simulink model "sar_adc_3"  (R2018a)
settings: Solver=ode23tb  StartTime=0.0  StopTime=1e-3  MaxStep=.5/ADC_clock  RelTol=1e-3  EnableMultiTasking=on
InitFcn:
  | % General Parameters
  | Nbits=12;
  | Fs=5e7;      % ADC conversion rate
  | ADC_clock = Fs*(Nbits+2); % required clock rate
  | 
  | 
  | % DAC parameters
  | Vref=2*sqrt(2);   % DAC voltage reference
  | Ron=100;             % switch on resistance
  | C=0.3e-12;           % unit capacitor
  | 
  | % Test Source Parameters
  | A1=Vref/4; A2=A1;   % amplitudes
  | F1=16*Fs/128;           % frequency
  | F2=18*Fs/128;
libraries: powerlib x64, simulink x26
settings Model: SimulationMode=accelerator  Creator=Dick  LastModifiedBy=lenovo
settings SolverCC: ZeroCrossControl=EnableAll  AlgebraicLoopSolver=LineSearch
settings DataIOCC: LimitDataPoints=on  SaveFormat=Array  SignalLoggingSaveFormat=ModelDataLogs
settings OptimizationCC: ExpressionDepthLimit=2147483647  LifeSpan=inf
settings DebuggingCC: UnderspecifiedInitializationDetection=Classic  MergeDetectMultiDrivingBlocksExec=none  SolverPrmCheckMsg=warning  ParameterPrecisionLossMsg=none  FcnCallInpInsideContextMsg=warning  StateNameClashWarn=warning  SFUnexpectedBacktrackingDiag=warning  SFNoUnconditionalDefaultTransitionDiag=warning  SFExecutionAtInitializationDiag=none
settings HardwareCC: ProdBitPerPointer=32  ProdBitPerSizeT=32  ProdBitPerPtrDiffT=32  ProdLargestAtomicFloat=None  ProdIntDivRoundTo=Undefined  ProdEndianess=Unspecified  ProdWordSize=32  ProdHWDeviceType=32-bit Generic
settings ModelReferenceCC: PropagateSignalLabelsOutOfModel=off
settings SFSimCC: SimParseCustomCode=off
settings CodeAppCC: StateflowObjectComments=on
settings GRTTargetCC: TargetLangStandard=C89/C90 (ANSI)  GeneratePreprocessorConditionals=Disable all  CombineOutputUpdateFcns=off  GRTInterface=on
settings ConfigComp: CovMetricSettings=dw  CovHtmlReporting=on  CovSaveCumulativeToWorkspaceVar=on  CovSaveSingleToWorkspaceVar=on  CovExternalEMLEnable=off  CovSFcnEnable=off
settings SimscapeCC: EditingMode=Restricted  SimscapeNormalizeSystem=off

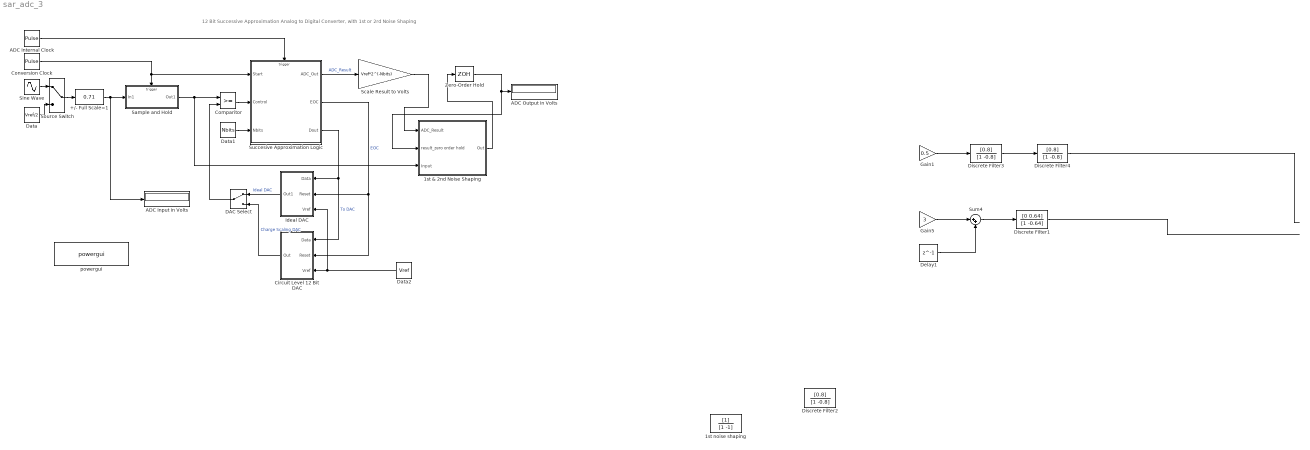
== system sar_adc_3 ==
  note: 12 Bit Successive Approximation Analog to Digital Converter, with 1st or 2rd Noise Shaping
  +/- Full Scale=1 : simulink/Math Operations/Slider Gain  gain=0.71  low=-1  high=1
  1st & 2nd Noise Shaping : Subsystem
  1st noise shaping : DiscreteFilter  Denominator=[1 -1]
  ADC Input in Volts : Display
      settings: Decimation=1000
  ADC Internal Clock : DiscretePulseGenerator  PulseType=Time based  Period=1/ADC_clock  PulseWidth=5
  ADC Output in Volts : Display
      settings: Decimation=1000
  Circuit Level 12 Bit DAC : Subsystem
  Comparitor : RelationalOperator  OutDataTypeStr=boolean  RndMeth=Nearest
  Conversion Clock : DiscretePulseGenerator  PulseType=Time based  Period=1/Fs  PulseWidth=5
  DAC Select : ManualSwitch
  Data : Constant  Value=Vref/2
  Data1 : Constant  Value=Nbits
  Data2 : Constant  Value=Vref
  Delay1 : Delay  DelayLength=1
  Discrete Filter1 : DiscreteFilter  Numerator=[0 0.64]  Denominator=[1 -0.64]
  Discrete Filter2 : DiscreteFilter  Numerator=[0.8]  Denominator=[1 -0.8]
  Discrete Filter3 : DiscreteFilter  Numerator=[0.8]  Denominator=[1 -0.8]
  Discrete Filter4 : DiscreteFilter  Numerator=[0.8]  Denominator=[1 -0.8]
  Gain1 : Gain  Gain=0.5
  Gain5 : Gain  Gain=3
  Ideal DAC : Subsystem
  Sample and Hold : Subsystem  TreatAsAtomicUnit=on
  Scale Result to Volts : Gain  Gain=Vref*2^(-Nbits)  OutDataTypeStr=double
  Sine Wave : Sin  Amplitude=2*A1  Frequency=2*pi*F1/5  SampleTime=0
  Source Switch : ManualSwitch
  Succesive Approximation Logic : Stateflow chart  TreatAsAtomicUnit=on
  Sum4 : Sum  Inputs=|++
  Zero-Order Hold : ZeroOrderHold  SampleTime=1/Fs
  powergui : powerlib/powergui  Priority=1  SimulationMode=Continuous  SampleTime=50e-6  frequency=60  Iterations=50  frequencyindice=0  Pbase=100e6  ErrMax=1e-4  UnitsV=kV  UnitsW=MW  buscounter=0  FunctionMessages=off  echomessages=off  EnableUseOfTLC=off  CurrentSourceSwitches=off  DisableSnubberDevices=on  DisableRonSwitches=off  DisableVfSwitches=off  DisplayEquations=off  SolverType=Tustin  Interpol=off  ExternalGateDelay=off  methode=off  Ts=0  x0status=blocks  SPID=on  SwTol=0  HookPort=off  RestoreLinks=warning  ResistiveCurrentMeasurement=off  Frange=[0:2:500]  Ylog=off  Xlog=on  ShowGrid=off  save=off  variable=ZData  structure=0  ZoomFFT=on  StartTime=0.0  cycles=1  DisplayStyle=1  fundamental=60  FreqAxis=off  MaxFrequency=1000  frequencyindicesteady=1  RmsSteady=1  display=off
  wires:
  ADC Internal Clock/1 -> Succesive Approximation Logic/Trigger
  Conversion Clock/1 -> Succesive Approximation Logic/1(Start), Sample and Hold/Trigger
  Succesive Approximation Logic/3(Dout) -> Circuit Level 12 Bit DAC/1(Data), Ideal DAC/1(Data)  "To DAC"
  Comparitor/1 -> Succesive Approximation Logic/2(Control)
  Succesive Approximation Logic/1(ADC_Out) -> Scale Result to Volts/1  "ADC_Result"
  Data1/1 -> Succesive Approximation Logic/3(Nbits)
  Data2/1 -> Circuit Level 12 Bit DAC/3(Vref), Ideal DAC/3(Vref)
  Circuit Level 12 Bit DAC/1(Out) -> DAC Select/2  "Charge Scaling DAC"
  Ideal DAC/1(Out1) -> DAC Select/1  "Ideal DAC"
  Zero-Order Hold/1 -> 1st & 2nd Noise Shaping/2(result_zero order hold), ADC Output in Volts/1
  Sine Wave/1 -> Source Switch/1
  +/- Full Scale=1/1 -> Sample and Hold/1(In1), ADC Input in Volts/1
  Source Switch/1 -> +/- Full Scale=1/1
  Succesive Approximation Logic/2(EOC) -> Ideal DAC/2(Reset), Circuit Level 12 Bit DAC/2(Reset)  "EOC"
  Data/1 -> Source Switch/2
  DAC Select/1 -> Comparitor/2
  Sample and Hold/1(Out1) -> Comparitor/1, 1st & 2nd Noise Shaping/3(Input)
  Discrete Filter3/1 -> Discrete Filter4/1
  ? -> Gain5/1
  Delay1/1 -> Sum4/2
  Gain1/1 -> Discrete Filter3/1
  ? -> Delay1/1
  Gain5/1 -> Sum4/1
  Sum4/1 -> Discrete Filter1/1
  Discrete Filter4/1 -> ?
  ? -> Gain1/1
  Discrete Filter1/1 -> ?
  Scale Result to Volts/1 -> 1st & 2nd Noise Shaping/1(ADC_Result)
  1st & 2nd Noise Shaping/1(Out) -> Zero-Order Hold/1

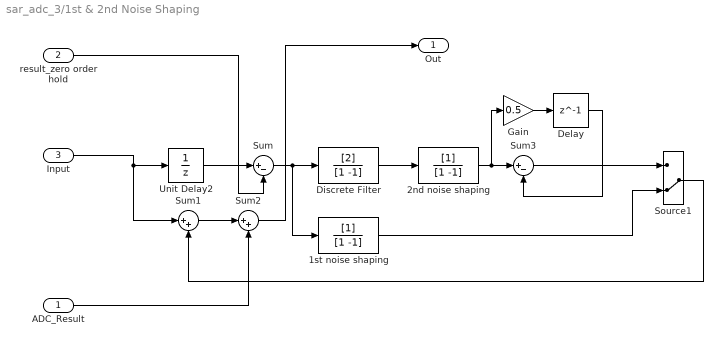
== system sar_adc_3/1st & 2nd Noise Shaping ==
  ADC_Result : Inport
  result_zero order hold : Inport  Port=2
  Input : Inport  Port=3
  1st noise shaping : DiscreteFilter  Denominator=[1 -1]
  2nd noise shaping : DiscreteFilter  Denominator=[1 -1]
  Delay : Delay  DelayLength=1
  Discrete Filter : DiscreteFilter  Numerator=[2]  Denominator=[1 -1]
  Gain : Gain  Gain=0.5
  Source1 : ManualSwitch  CurrentSetting=0
  Sum : Sum  Inputs=|+-
  Sum1 : Sum  Inputs=|++
  Sum2 : Sum  Inputs=|++
  Sum3 : Sum  Inputs=|+-
  Unit Delay2 : UnitDelay  SampleTime=1/Fs
  Out : Outport
  wires:
  Delay/1 -> Sum3/2
  Input/1 -> Sum1/1, Unit Delay2/1
  Sum3/1 -> Source1/1
  2nd noise shaping/1 -> Gain/1, Sum3/1
  Gain/1 -> Delay/1
  Discrete Filter/1 -> 2nd noise shaping/1
  1st noise shaping/1 -> Source1/2
  Sum1/1 -> Sum2/1
  Unit Delay2/1 -> Sum/1
  Source1/1 -> Sum1/2
  Sum/1 -> Discrete Filter/1, 1st noise shaping/1
  Sum2/1 -> Out/1
  result_zero order hold/1 -> Sum/2
  ADC_Result/1 -> Sum2/2

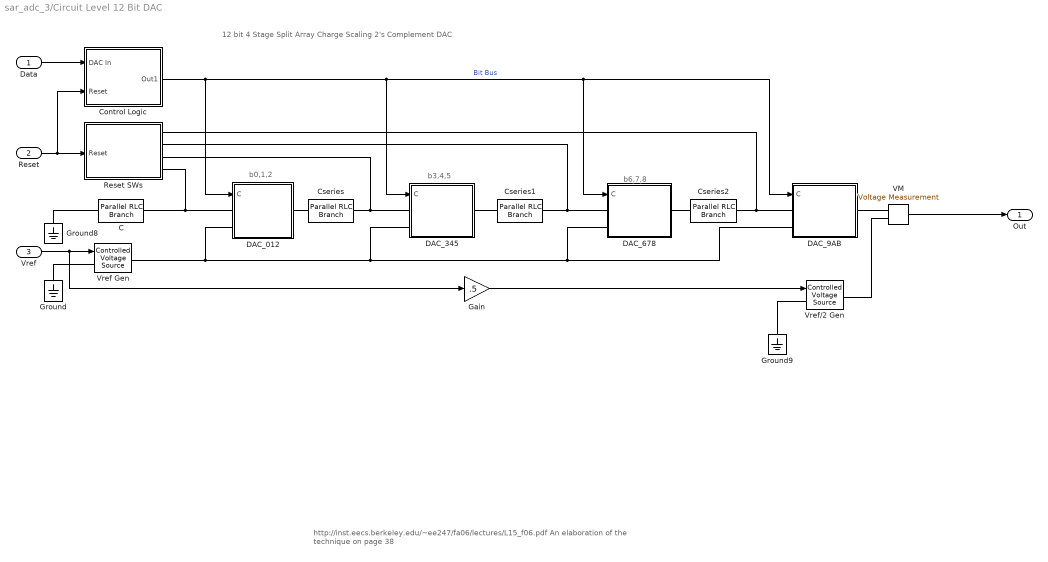
== system sar_adc_3/Circuit Level 12 Bit DAC ==
  note: http://inst.eecs.berkeley.edu/~ee247/fa06/lectures/L15_f06.pdf
      | An elaboration of the technique on page 38
  note: b6,7,8
  note: b3,4,5
  note: b0,1,2
  note: 12 bit 4 Stage Split Array Charge Scaling 2's Complement DAC
  Data : Inport
  Reset : Inport  Port=2
  Vref : Inport  Port=3
  C : powerlib/Elements/Parallel RLC Branch  LConnTagsString=a  RConnTagsString=__new0  BranchType=C  Resistance=1  Inductance=1e-3  SetiL0=off  InitialCurrent=0  Capacitance=C  Setx0=off  InitialVoltage=0  Measurements=None
  Control Logic : Subsystem
  Cseries : powerlib/Elements/Parallel RLC Branch  LConnTagsString=a  RConnTagsString=__new0  BranchType=C  Resistance=1  Inductance=1e-3  SetiL0=off  InitialCurrent=0  Capacitance=C*8/7  Setx0=off  InitialVoltage=0  Measurements=None
  Cseries1 : powerlib/Elements/Parallel RLC Branch  LConnTagsString=a  RConnTagsString=__new0  BranchType=C  Resistance=1  Inductance=1e-3  SetiL0=off  InitialCurrent=0  Capacitance=C*8/7  Setx0=off  InitialVoltage=0  Measurements=None
  Cseries2 : powerlib/Elements/Parallel RLC Branch  LConnTagsString=a  RConnTagsString=__new0  BranchType=C  Resistance=1  Inductance=1e-3  SetiL0=off  InitialCurrent=0  Capacitance=C*8/7  Setx0=off  InitialVoltage=0  Measurements=None
  DAC_012 : Subsystem
  DAC_345 : Subsystem
  DAC_678 : Subsystem
  DAC_9AB : Subsystem
  Gain : Gain  Gain=.5
  Ground : powerlib/Elements/Ground  LConnTagsString=a
  Ground8 : powerlib/Elements/Ground  LConnTagsString=a
  Ground9 : powerlib/Elements/Ground  LConnTagsString=a
  Reset SWs : Subsystem
  VM : powerlib/Measurements/Voltage Measurement  PhasorSimulation=off  OutputType=Complex  PSBequivalent=0
  Vref Gen : powerlib/Electrical Sources/Controlled Voltage Source  Initialize=off  Source_Type=DC  Amplitude=0  Phase=0  Frequency=0  Measurements=None
  Vref/2 Gen : powerlib/Electrical Sources/Controlled Voltage Source  Initialize=off  Source_Type=DC  Amplitude=0  Phase=0  Frequency=0  Measurements=None
  Out : Outport
  wires:
  Vref/1 -> Vref Gen/1, Gain/1
  Data/1 -> Control Logic/1(DAC In)
  Control Logic/1(Out1) -> DAC_9AB/1(C), DAC_678/1(C), DAC_345/1(C), DAC_012/1(C)  "Bit Bus"
  VM/1 -> Out/1
  Reset/1 -> Reset SWs/1(Reset), Control Logic/2(Reset)
  Gain/1 -> Vref/2 Gen/1
  connections:
  Vref Gen/LConn1 -- Ground/LConn1
  VM/LConn1 -- DAC_9AB/RConn1
  DAC_9AB/LConn2 -- DAC_678/LConn2 -- DAC_345/LConn2 -- Vref Gen/RConn1 -- DAC_012/LConn2
  DAC_678/RConn1 -- Cseries2/RConn1
  DAC_9AB/LConn1 -- Reset SWs/RConn1 -- Cseries2/LConn1
  Cseries1/RConn1 -- DAC_345/RConn1
  DAC_678/LConn1 -- Reset SWs/RConn2 -- Cseries1/LConn1
  Cseries/RConn1 -- DAC_012/RConn1
  Reset SWs/RConn3 -- DAC_345/LConn1 -- Cseries/LConn1
  Ground8/LConn1 -- C/RConn1
  DAC_012/LConn1 -- Reset SWs/RConn4 -- C/LConn1
  Vref/2 Gen/RConn1 -- VM/LConn2
  Vref/2 Gen/LConn1 -- Ground9/LConn1

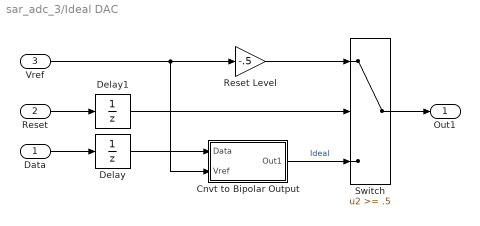
== system sar_adc_3/Ideal DAC ==
  Data : Inport
  Reset : Inport  Port=2
  Vref : Inport  Port=3
  Cnvt to Bipolar Output : Subsystem
  Delay : UnitDelay  SampleTime=1/ADC_clock
  Delay1 : UnitDelay  SampleTime=1/ADC_clock
  Reset Level : Gain  Gain=-.5
  Switch : Switch  Threshold=.5
  Out1 : Outport
  wires:
  Delay/1 -> Cnvt to Bipolar Output/1(Data)
  Data/1 -> Delay/1
  Vref/1 -> Cnvt to Bipolar Output/2(Vref), Reset Level/1
  Reset/1 -> Delay1/1
  Cnvt to Bipolar Output/1(Out1) -> Switch/3  "Ideal"
  Switch/1 -> Out1/1
  Reset Level/1 -> Switch/1
  Delay1/1 -> Switch/2

== system sar_adc_3/Sample and Hold ==
  In1 : Inport
  Trigger : TriggerPort  VariantControl=(inherit)
  Out1 : Outport
  wires:
  In1/1 -> Out1/1

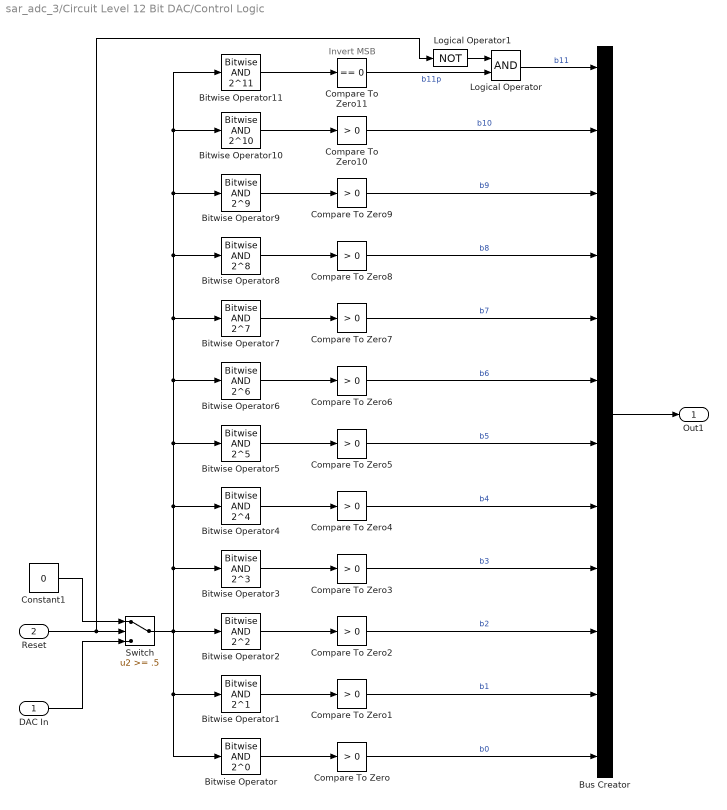
== system sar_adc_3/Circuit Level 12 Bit DAC/Control Logic ==
  note: Invert MSB
  DAC In : Inport
  Reset : Inport  Port=2
  Bitwise Operator : simulink/Logic and Bit Operations/Bitwise Operator  logicop=AND  UseBitMask=on  BitMask=2^0  BitMaskRealWorld=Stored Integer
  Bitwise Operator1 : simulink/Logic and Bit Operations/Bitwise Operator  logicop=AND  UseBitMask=on  BitMask=2^1  BitMaskRealWorld=Stored Integer
  Bitwise Operator10 : simulink/Logic and Bit Operations/Bitwise Operator  logicop=AND  UseBitMask=on  BitMask=2^10  BitMaskRealWorld=Stored Integer
  Bitwise Operator11 : simulink/Logic and Bit Operations/Bitwise Operator  logicop=AND  UseBitMask=on  BitMask=2^11  BitMaskRealWorld=Stored Integer
  Bitwise Operator2 : simulink/Logic and Bit Operations/Bitwise Operator  logicop=AND  UseBitMask=on  BitMask=2^2  BitMaskRealWorld=Stored Integer
  Bitwise Operator3 : simulink/Logic and Bit Operations/Bitwise Operator  logicop=AND  UseBitMask=on  BitMask=2^3  BitMaskRealWorld=Stored Integer
  Bitwise Operator4 : simulink/Logic and Bit Operations/Bitwise Operator  logicop=AND  UseBitMask=on  BitMask=2^4  BitMaskRealWorld=Stored Integer
  Bitwise Operator5 : simulink/Logic and Bit Operations/Bitwise Operator  logicop=AND  UseBitMask=on  BitMask=2^5  BitMaskRealWorld=Stored Integer
  Bitwise Operator6 : simulink/Logic and Bit Operations/Bitwise Operator  logicop=AND  UseBitMask=on  BitMask=2^6  BitMaskRealWorld=Stored Integer
  Bitwise Operator7 : simulink/Logic and Bit Operations/Bitwise Operator  logicop=AND  UseBitMask=on  BitMask=2^7  BitMaskRealWorld=Stored Integer
  Bitwise Operator8 : simulink/Logic and Bit Operations/Bitwise Operator  logicop=AND  UseBitMask=on  BitMask=2^8  BitMaskRealWorld=Stored Integer
  Bitwise Operator9 : simulink/Logic and Bit Operations/Bitwise Operator  logicop=AND  UseBitMask=on  BitMask=2^9  BitMaskRealWorld=Stored Integer
  Bus Creator : BusCreator  Inputs=12
  Compare To Zero{,1..10} (11 alike) : simulink/Logic and Bit Operations/Compare To Zero  relop=>  OutDataTypeStr=boolean
  Compare To Zero11 : simulink/Logic and Bit Operations/Compare To Zero  relop===  OutDataTypeStr=boolean
  Constant1 : Constant  Value=0  OutDataTypeStr=int16
  Logical Operator : Logic  AllPortsSameDT=off  OutDataTypeStr=boolean
  Logical Operator1 : Logic  Operator=NOT  AllPortsSameDT=off  OutDataTypeStr=boolean
  Switch : Switch  Threshold=.5
  Out1 : Outport
  wires:
  Compare To Zero10/1 -> Bus Creator/2  "b10"
  Bitwise Operator11/1 -> Compare To Zero11/1
  Bitwise Operator10/1 -> Compare To Zero10/1
  Compare To Zero9/1 -> Bus Creator/3  "b9"
  Bitwise Operator9/1 -> Compare To Zero9/1
  Compare To Zero8/1 -> Bus Creator/4  "b8"
  Compare To Zero7/1 -> Bus Creator/5  "b7"
  Compare To Zero6/1 -> Bus Creator/6  "b6"
  Compare To Zero5/1 -> Bus Creator/7  "b5"
  Compare To Zero4/1 -> Bus Creator/8  "b4"
  Compare To Zero3/1 -> Bus Creator/9  "b3"
  Compare To Zero2/1 -> Bus Creator/10  "b2"
  Compare To Zero1/1 -> Bus Creator/11  "b1"
  Compare To Zero/1 -> Bus Creator/12  "b0"
  Bitwise Operator8/1 -> Compare To Zero8/1
  Bitwise Operator7/1 -> Compare To Zero7/1
  Bitwise Operator6/1 -> Compare To Zero6/1
  Bitwise Operator5/1 -> Compare To Zero5/1
  Bitwise Operator4/1 -> Compare To Zero4/1
  Reset/1 -> Switch/2, Logical Operator1/1
  Constant1/1 -> Switch/1
  DAC In/1 -> Switch/3
  Switch/1 -> Bitwise Operator10/1, Bitwise Operator11/1, Bitwise Operator9/1, Bitwise Operator8/1, Bitwise Operator7/1, Bitwise Operator6/1, Bitwise Operator5/1, Bitwise Operator4/1, Bitwise Operator3/1, Bitwise Operator1/1, Bitwise Operator/1, Bitwise Operator2/1
  Bus Creator/1 -> Out1/1
  Bitwise Operator3/1 -> Compare To Zero3/1
  Bitwise Operator2/1 -> Compare To Zero2/1
  Bitwise Operator1/1 -> Compare To Zero1/1
  Bitwise Operator/1 -> Compare To Zero/1
  Logical Operator/1 -> Bus Creator/1  "b11"
  Compare To Zero11/1 -> Logical Operator/2  "b11p"
  Logical Operator1/1 -> Logical Operator/1

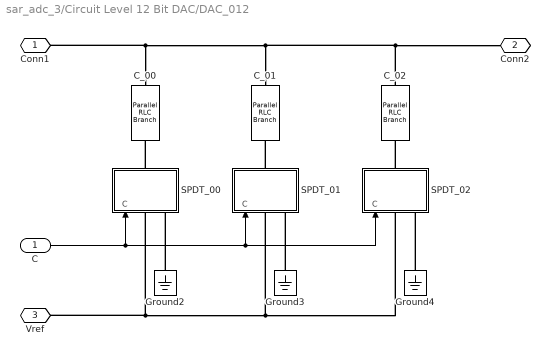
== system sar_adc_3/Circuit Level 12 Bit DAC/DAC_012 ==
  C : Inport
  C_00 : powerlib/Elements/Parallel RLC Branch  LConnTagsString=a  RConnTagsString=__new0  BranchType=C  Resistance=1  Inductance=1e-3  SetiL0=off  InitialCurrent=0  Capacitance=C  Setx0=off  InitialVoltage=0  Measurements=None
  C_01 : powerlib/Elements/Parallel RLC Branch  LConnTagsString=a  RConnTagsString=__new0  BranchType=C  Resistance=1  Inductance=1e-3  SetiL0=off  InitialCurrent=0  Capacitance=C*2^1  Setx0=off  InitialVoltage=0  Measurements=None
  C_02 : powerlib/Elements/Parallel RLC Branch  LConnTagsString=a  RConnTagsString=__new0  BranchType=C  Resistance=1  Inductance=1e-3  SetiL0=off  InitialCurrent=0  Capacitance=C*2^2  Setx0=off  InitialVoltage=0  Measurements=None
  Ground2 : powerlib/Elements/Ground  LConnTagsString=a
  Ground3 : powerlib/Elements/Ground  LConnTagsString=a
  Ground4 : powerlib/Elements/Ground  LConnTagsString=a
  SPDT_00 : Subsystem
  SPDT_01 : Subsystem
  SPDT_02 : Subsystem
  Conn1 : PMIOPort  Side=Left
  Conn2 : PMIOPort  Port=2  Side=Right
  Vref : PMIOPort  Port=3  Side=Left
  wires:
  C/1 -> SPDT_01/1(C), SPDT_02/1(C), SPDT_00/1(C)
  connections:
  SPDT_00/LConn1 -- SPDT_02/LConn1 -- SPDT_01/LConn1 -- Vref/RConn1
  Ground4/LConn1 -- SPDT_02/LConn2
  Ground3/LConn1 -- SPDT_01/LConn2
  Ground2/LConn1 -- SPDT_00/LConn2
  SPDT_02/RConn1 -- C_02/RConn1
  SPDT_01/RConn1 -- C_01/RConn1
  SPDT_00/RConn1 -- C_00/RConn1
  Conn1/RConn1 -- C_00/LConn1 -- C_01/LConn1 -- C_02/LConn1 -- Conn2/RConn1

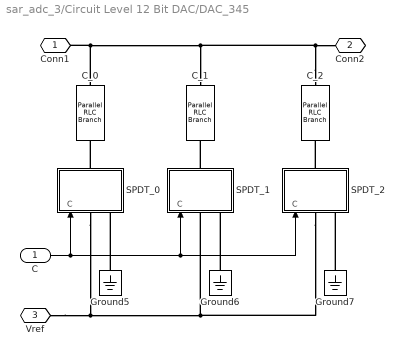
== system sar_adc_3/Circuit Level 12 Bit DAC/DAC_345 ==
  C : Inport
  C_0 : powerlib/Elements/Parallel RLC Branch  LConnTagsString=a  RConnTagsString=__new0  BranchType=C  Resistance=1  Inductance=1e-3  SetiL0=off  InitialCurrent=0  Capacitance=C*2^0  Setx0=off  InitialVoltage=0  Measurements=None
  C_1 : powerlib/Elements/Parallel RLC Branch  LConnTagsString=a  RConnTagsString=__new0  BranchType=C  Resistance=1  Inductance=1e-3  SetiL0=off  InitialCurrent=0  Capacitance=C*2^1  Setx0=off  InitialVoltage=0  Measurements=None
  C_2 : powerlib/Elements/Parallel RLC Branch  LConnTagsString=a  RConnTagsString=__new0  BranchType=C  Resistance=1  Inductance=1e-3  SetiL0=off  InitialCurrent=0  Capacitance=C*2^2  Setx0=off  InitialVoltage=0  Measurements=None
  Ground5 : powerlib/Elements/Ground  LConnTagsString=a
  Ground6 : powerlib/Elements/Ground  LConnTagsString=a
  Ground7 : powerlib/Elements/Ground  LConnTagsString=a
  SPDT_0 : Subsystem
  SPDT_1 : Subsystem
  SPDT_2 : Subsystem
  Conn1 : PMIOPort  Side=Left
  Conn2 : PMIOPort  Port=2  Side=Right
  Vref : PMIOPort  Port=3  Side=Left
  wires:
  C/1 -> SPDT_2/1(C), SPDT_1/1(C), SPDT_0/1(C)
  connections:
  Vref/RConn1 -- SPDT_0/LConn1 -- SPDT_1/LConn1 -- SPDT_2/LConn1
  Ground7/LConn1 -- SPDT_2/LConn2
  Ground6/LConn1 -- SPDT_1/LConn2
  Ground5/LConn1 -- SPDT_0/LConn2
  SPDT_2/RConn1 -- C_2/RConn1
  SPDT_1/RConn1 -- C_1/RConn1
  SPDT_0/RConn1 -- C_0/RConn1
  C_2/LConn1 -- C_1/LConn1 -- Conn1/RConn1 -- C_0/LConn1 -- Conn2/RConn1

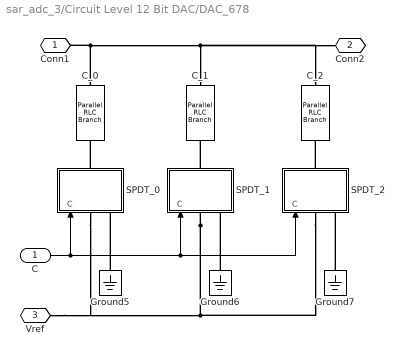
== system sar_adc_3/Circuit Level 12 Bit DAC/DAC_678 ==
  C : Inport
  C_0 : powerlib/Elements/Parallel RLC Branch  LConnTagsString=a  RConnTagsString=__new0  BranchType=C  Resistance=1  Inductance=1e-3  SetiL0=off  InitialCurrent=0  Capacitance=C*2^0  Setx0=off  InitialVoltage=0  Measurements=None
  C_1 : powerlib/Elements/Parallel RLC Branch  LConnTagsString=a  RConnTagsString=__new0  BranchType=C  Resistance=1  Inductance=1e-3  SetiL0=off  InitialCurrent=0  Capacitance=C*2^1  Setx0=off  InitialVoltage=0  Measurements=None
  C_2 : powerlib/Elements/Parallel RLC Branch  LConnTagsString=a  RConnTagsString=__new0  BranchType=C  Resistance=1  Inductance=1e-3  SetiL0=off  InitialCurrent=0  Capacitance=C*2^2  Setx0=off  InitialVoltage=0  Measurements=None
  Ground5 : powerlib/Elements/Ground  LConnTagsString=a
  Ground6 : powerlib/Elements/Ground  LConnTagsString=a
  Ground7 : powerlib/Elements/Ground  LConnTagsString=a
  SPDT_0 : Subsystem
  SPDT_1 : Subsystem
  SPDT_2 : Subsystem
  Conn1 : PMIOPort  Side=Left
  Conn2 : PMIOPort  Port=2  Side=Right
  Vref : PMIOPort  Port=3  Side=Left
  wires:
  C/1 -> SPDT_0/1(C), SPDT_1/1(C), SPDT_2/1(C)
  connections:
  C_0/LConn1 -- Conn1/RConn1 -- C_1/LConn1 -- Conn2/RConn1 -- C_2/LConn1
  SPDT_0/RConn1 -- C_0/RConn1
  SPDT_1/RConn1 -- C_1/RConn1
  SPDT_2/RConn1 -- C_2/RConn1
  Ground5/LConn1 -- SPDT_0/LConn2
  Ground6/LConn1 -- SPDT_1/LConn2
  Ground7/LConn1 -- SPDT_2/LConn2
  SPDT_1/LConn1 -- SPDT_0/LConn1 -- Vref/RConn1 -- SPDT_2/LConn1

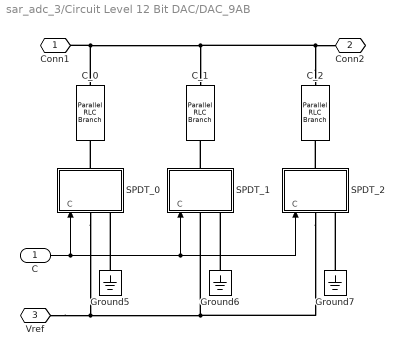
== system sar_adc_3/Circuit Level 12 Bit DAC/DAC_9AB ==
  C : Inport
  C_0 : powerlib/Elements/Parallel RLC Branch  LConnTagsString=a  RConnTagsString=__new0  BranchType=C  Resistance=1  Inductance=1e-3  SetiL0=off  InitialCurrent=0  Capacitance=C*2^0  Setx0=off  InitialVoltage=0  Measurements=None
  C_1 : powerlib/Elements/Parallel RLC Branch  LConnTagsString=a  RConnTagsString=__new0  BranchType=C  Resistance=1  Inductance=1e-3  SetiL0=off  InitialCurrent=0  Capacitance=C*2^1  Setx0=off  InitialVoltage=0  Measurements=None
  C_2 : powerlib/Elements/Parallel RLC Branch  LConnTagsString=a  RConnTagsString=__new0  BranchType=C  Resistance=1  Inductance=1e-3  SetiL0=off  InitialCurrent=0  Capacitance=C*2^2  Setx0=off  InitialVoltage=0  Measurements=None
  Ground5 : powerlib/Elements/Ground  LConnTagsString=a
  Ground6 : powerlib/Elements/Ground  LConnTagsString=a
  Ground7 : powerlib/Elements/Ground  LConnTagsString=a
  SPDT_0 : Subsystem
  SPDT_1 : Subsystem
  SPDT_2 : Subsystem
  Conn1 : PMIOPort  Side=Left
  Conn2 : PMIOPort  Port=2  Side=Right
  Vref : PMIOPort  Port=3  Side=Left
  wires:
  C/1 -> SPDT_2/1(C), SPDT_1/1(C), SPDT_0/1(C)
  connections:
  SPDT_2/LConn1 -- SPDT_0/LConn1 -- Vref/RConn1 -- SPDT_1/LConn1
  Ground7/LConn1 -- SPDT_2/LConn2
  Ground6/LConn1 -- SPDT_1/LConn2
  Ground5/LConn1 -- SPDT_0/LConn2
  SPDT_2/RConn1 -- C_2/RConn1
  SPDT_1/RConn1 -- C_1/RConn1
  SPDT_0/RConn1 -- C_0/RConn1
  C_2/LConn1 -- Conn2/RConn1 -- C_1/LConn1 -- Conn1/RConn1 -- C_0/LConn1

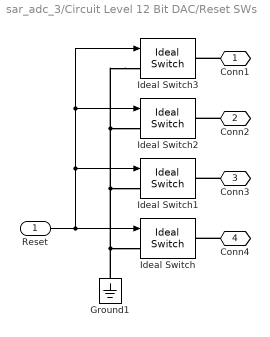
== system sar_adc_3/Circuit Level 12 Bit DAC/Reset SWs ==
  Reset : Inport
  Ground1 : powerlib/Elements/Ground  LConnTagsString=a
  Ideal Switch{,1..3} (4 alike) : powerlib/Power Electronics/Ideal Switch  Ron=Ron  Lon=0  IC=0  Rs=inf  Cs=0  Measurements=off
  Conn1 : PMIOPort  Side=Right
  Conn2 : PMIOPort  Port=2  Side=Right
  Conn3 : PMIOPort  Port=3  Side=Right
  Conn4 : PMIOPort  Port=4  Side=Right
  wires:
  Reset/1 -> Ideal Switch2/1, Ideal Switch3/1, Ideal Switch1/1, Ideal Switch/1
  connections:
  Conn4/RConn1 -- Ideal Switch/RConn1
  Conn3/RConn1 -- Ideal Switch1/RConn1
  Conn2/RConn1 -- Ideal Switch2/RConn1
  Conn1/RConn1 -- Ideal Switch3/RConn1
  Ideal Switch3/LConn1 -- Ideal Switch2/LConn1 -- Ideal Switch1/LConn1 -- Ideal Switch/LConn1 -- Ground1/LConn1

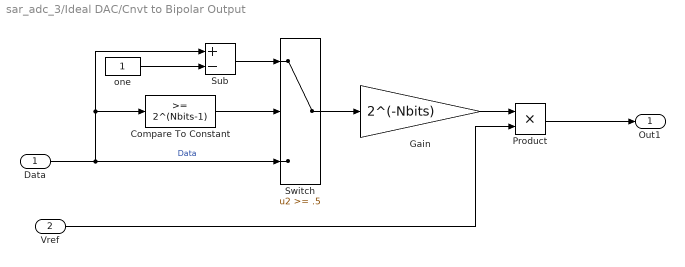
== system sar_adc_3/Ideal DAC/Cnvt to Bipolar Output ==
  Data : Inport
  Vref : Inport  Port=2
  Compare To Constant : simulink/Logic and Bit Operations/Compare To Constant  relop=>=  const=2^(Nbits-1)  OutDataTypeStr=boolean
  Gain : Gain  Gain=2^(-Nbits)
  Product : Product  RndMeth=Zero
  Sub : Sum  Inputs=+-  OutDataTypeStr=double
  Switch : Switch  Threshold=.5
  one : Constant  OutDataTypeStr=int16
  Out1 : Outport
  wires:
  one/1 -> Sub/2
  Compare To Constant/1 -> Switch/2
  Sub/1 -> Switch/1
  Switch/1 -> Gain/1
  Data/1 -> Switch/3, Sub/1, Compare To Constant/1  "Data"
  Gain/1 -> Product/1
  Product/1 -> Out1/1
  Vref/1 -> Product/2

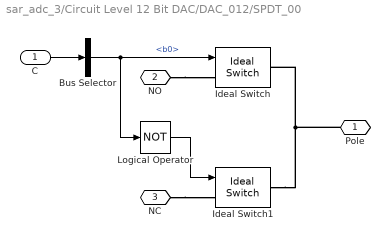
== system sar_adc_3/Circuit Level 12 Bit DAC/DAC_012/SPDT_00 ==
  C : Inport
  Bus Selector : BusSelector  OutputSignals=b0
  Ideal Switch : powerlib/Power Electronics/Ideal Switch  Ron=Ron  Lon=0  IC=0  Rs=inf  Cs=0  Measurements=off
  Ideal Switch1 : powerlib/Power Electronics/Ideal Switch  Ron=Ron  Lon=0  IC=0  Rs=inf  Cs=0  Measurements=off
  Logical Operator : Logic  Operator=NOT  AllPortsSameDT=off  OutDataTypeStr=boolean
  Pole : PMIOPort  Side=Right
  NO : PMIOPort  Port=2  Side=Left
  NC : PMIOPort  Port=3  Side=Left
  wires:
  Bus Selector/1 -> Ideal Switch/1, Logical Operator/1  "<b0>"
  Logical Operator/1 -> Ideal Switch1/1
  C/1 -> Bus Selector/1
  connections:
  Ideal Switch1/RConn1 -- Pole/RConn1 -- Ideal Switch/RConn1
  NO/RConn1 -- Ideal Switch/LConn1
  NC/RConn1 -- Ideal Switch1/LConn1

== system sar_adc_3/Circuit Level 12 Bit DAC/DAC_012/SPDT_01 ==
  C : Inport
  Bus Selector : BusSelector  OutputSignals=b1
  Ideal Switch : powerlib/Power Electronics/Ideal Switch  Ron=Ron  Lon=0  IC=0  Rs=inf  Cs=0  Measurements=off
  Ideal Switch1 : powerlib/Power Electronics/Ideal Switch  Ron=Ron  Lon=0  IC=0  Rs=inf  Cs=0  Measurements=off
  Logical Operator : Logic  Operator=NOT  AllPortsSameDT=off  OutDataTypeStr=boolean
  Pole : PMIOPort  Side=Right
  NO : PMIOPort  Port=2  Side=Left
  NC : PMIOPort  Port=3  Side=Left
  wires:
  Bus Selector/1 -> Logical Operator/1, Ideal Switch/1  "<b1>"
  C/1 -> Bus Selector/1
  Logical Operator/1 -> Ideal Switch1/1
  connections:
  NC/RConn1 -- Ideal Switch1/LConn1
  NO/RConn1 -- Ideal Switch/LConn1
  Ideal Switch/RConn1 -- Pole/RConn1 -- Ideal Switch1/RConn1

== system sar_adc_3/Circuit Level 12 Bit DAC/DAC_012/SPDT_02 ==
  C : Inport
  Bus Selector : BusSelector  OutputSignals=b2
  Ideal Switch : powerlib/Power Electronics/Ideal Switch  Ron=Ron  Lon=0  IC=0  Rs=inf  Cs=0  Measurements=off
  Ideal Switch1 : powerlib/Power Electronics/Ideal Switch  Ron=Ron  Lon=0  IC=0  Rs=inf  Cs=0  Measurements=off
  Logical Operator : Logic  Operator=NOT  AllPortsSameDT=off  OutDataTypeStr=boolean
  Pole : PMIOPort  Side=Right
  NO : PMIOPort  Port=2  Side=Left
  NC : PMIOPort  Port=3  Side=Left
  wires:
  Bus Selector/1 -> Ideal Switch/1, Logical Operator/1  "<b2>"
  Logical Operator/1 -> Ideal Switch1/1
  C/1 -> Bus Selector/1
  connections:
  Ideal Switch1/RConn1 -- Pole/RConn1 -- Ideal Switch/RConn1
  NO/RConn1 -- Ideal Switch/LConn1
  NC/RConn1 -- Ideal Switch1/LConn1

== system sar_adc_3/Circuit Level 12 Bit DAC/DAC_345/SPDT_0 ==
  C : Inport
  Bus Selector : BusSelector  OutputSignals=b3
  Ideal Switch : powerlib/Power Electronics/Ideal Switch  Ron=Ron  Lon=0  IC=0  Rs=inf  Cs=0  Measurements=off
  Ideal Switch1 : powerlib/Power Electronics/Ideal Switch  Ron=Ron  Lon=0  IC=0  Rs=inf  Cs=0  Measurements=off
  Logical Operator : Logic  Operator=NOT  AllPortsSameDT=off  OutDataTypeStr=boolean
  Pole : PMIOPort  Side=Right
  NO : PMIOPort  Port=2  Side=Left
  NC : PMIOPort  Port=3  Side=Left
  wires:
  Bus Selector/1 -> Logical Operator/1, Ideal Switch/1  "<b3>"
  C/1 -> Bus Selector/1
  Logical Operator/1 -> Ideal Switch1/1
  connections:
  NC/RConn1 -- Ideal Switch1/LConn1
  NO/RConn1 -- Ideal Switch/LConn1
  Ideal Switch1/RConn1 -- Ideal Switch/RConn1 -- Pole/RConn1

== system sar_adc_3/Circuit Level 12 Bit DAC/DAC_345/SPDT_1 ==
  C : Inport
  Bus Selector : BusSelector  OutputSignals=b4
  Ideal Switch : powerlib/Power Electronics/Ideal Switch  Ron=Ron  Lon=0  IC=0  Rs=inf  Cs=0  Measurements=off
  Ideal Switch1 : powerlib/Power Electronics/Ideal Switch  Ron=Ron  Lon=0  IC=0  Rs=inf  Cs=0  Measurements=off
  Logical Operator : Logic  Operator=NOT  AllPortsSameDT=off  OutDataTypeStr=boolean
  Pole : PMIOPort  Side=Right
  NO : PMIOPort  Port=2  Side=Left
  NC : PMIOPort  Port=3  Side=Left
  wires:
  Logical Operator/1 -> Ideal Switch1/1
  C/1 -> Bus Selector/1
  Bus Selector/1 -> Ideal Switch/1, Logical Operator/1  "<b4>"
  connections:
  Pole/RConn1 -- Ideal Switch/RConn1 -- Ideal Switch1/RConn1
  NO/RConn1 -- Ideal Switch/LConn1
  NC/RConn1 -- Ideal Switch1/LConn1

== system sar_adc_3/Circuit Level 12 Bit DAC/DAC_345/SPDT_2 ==
  C : Inport
  Bus Selector : BusSelector  OutputSignals=b5
  Ideal Switch : powerlib/Power Electronics/Ideal Switch  Ron=Ron  Lon=0  IC=0  Rs=inf  Cs=0  Measurements=off
  Ideal Switch1 : powerlib/Power Electronics/Ideal Switch  Ron=Ron  Lon=0  IC=0  Rs=inf  Cs=0  Measurements=off
  Logical Operator : Logic  Operator=NOT  AllPortsSameDT=off  OutDataTypeStr=boolean
  Pole : PMIOPort  Side=Right
  NO : PMIOPort  Port=2  Side=Left
  NC : PMIOPort  Port=3  Side=Left
  wires:
  Bus Selector/1 -> Logical Operator/1, Ideal Switch/1  "<b5>"
  C/1 -> Bus Selector/1
  Logical Operator/1 -> Ideal Switch1/1
  connections:
  NC/RConn1 -- Ideal Switch1/LConn1
  NO/RConn1 -- Ideal Switch/LConn1
  Ideal Switch1/RConn1 -- Ideal Switch/RConn1 -- Pole/RConn1

== system sar_adc_3/Circuit Level 12 Bit DAC/DAC_678/SPDT_0 ==
  C : Inport
  Bus Selector : BusSelector  OutputSignals=b6
  Ideal Switch : powerlib/Power Electronics/Ideal Switch  Ron=Ron  Lon=0  IC=0  Rs=inf  Cs=0  Measurements=off
  Ideal Switch1 : powerlib/Power Electronics/Ideal Switch  Ron=Ron  Lon=0  IC=0  Rs=inf  Cs=0  Measurements=off
  Logical Operator : Logic  Operator=NOT  AllPortsSameDT=off  OutDataTypeStr=boolean
  Pole : PMIOPort  Side=Right
  NO : PMIOPort  Port=2  Side=Left
  NC : PMIOPort  Port=3  Side=Left
  wires:
  Logical Operator/1 -> Ideal Switch1/1
  C/1 -> Bus Selector/1
  Bus Selector/1 -> Ideal Switch/1, Logical Operator/1  "<b6>"
  connections:
  Pole/RConn1 -- Ideal Switch/RConn1 -- Ideal Switch1/RConn1
  NO/RConn1 -- Ideal Switch/LConn1
  NC/RConn1 -- Ideal Switch1/LConn1

== system sar_adc_3/Circuit Level 12 Bit DAC/DAC_678/SPDT_1 ==
  C : Inport
  Bus Selector : BusSelector  OutputSignals=b7
  Ideal Switch : powerlib/Power Electronics/Ideal Switch  Ron=Ron  Lon=0  IC=0  Rs=inf  Cs=0  Measurements=off
  Ideal Switch1 : powerlib/Power Electronics/Ideal Switch  Ron=Ron  Lon=0  IC=0  Rs=inf  Cs=0  Measurements=off
  Logical Operator : Logic  Operator=NOT  AllPortsSameDT=off  OutDataTypeStr=boolean
  Pole : PMIOPort  Side=Right
  NO : PMIOPort  Port=2  Side=Left
  NC : PMIOPort  Port=3  Side=Left
  wires:
  Bus Selector/1 -> Logical Operator/1, Ideal Switch/1  "<b7>"
  C/1 -> Bus Selector/1
  Logical Operator/1 -> Ideal Switch1/1
  connections:
  NC/RConn1 -- Ideal Switch1/LConn1
  NO/RConn1 -- Ideal Switch/LConn1
  Ideal Switch1/RConn1 -- Ideal Switch/RConn1 -- Pole/RConn1

== system sar_adc_3/Circuit Level 12 Bit DAC/DAC_678/SPDT_2 ==
  C : Inport
  Bus Selector : BusSelector  OutputSignals=b8
  Ideal Switch : powerlib/Power Electronics/Ideal Switch  Ron=Ron  Lon=0  IC=0  Rs=inf  Cs=0  Measurements=off
  Ideal Switch1 : powerlib/Power Electronics/Ideal Switch  Ron=Ron  Lon=0  IC=0  Rs=inf  Cs=0  Measurements=off
  Logical Operator : Logic  Operator=NOT  AllPortsSameDT=off  OutDataTypeStr=boolean
  Pole : PMIOPort  Side=Right
  NO : PMIOPort  Port=2  Side=Left
  NC : PMIOPort  Port=3  Side=Left
  wires:
  Logical Operator/1 -> Ideal Switch1/1
  C/1 -> Bus Selector/1
  Bus Selector/1 -> Ideal Switch/1, Logical Operator/1  "<b8>"
  connections:
  Pole/RConn1 -- Ideal Switch/RConn1 -- Ideal Switch1/RConn1
  NO/RConn1 -- Ideal Switch/LConn1
  NC/RConn1 -- Ideal Switch1/LConn1

== system sar_adc_3/Circuit Level 12 Bit DAC/DAC_9AB/SPDT_0 ==
  C : Inport
  Bus Selector : BusSelector  OutputSignals=b9
  Ideal Switch : powerlib/Power Electronics/Ideal Switch  Ron=Ron  Lon=0  IC=0  Rs=inf  Cs=0  Measurements=off
  Ideal Switch1 : powerlib/Power Electronics/Ideal Switch  Ron=Ron  Lon=0  IC=0  Rs=inf  Cs=0  Measurements=off
  Logical Operator : Logic  Operator=NOT  AllPortsSameDT=off  OutDataTypeStr=boolean
  Pole : PMIOPort  Side=Right
  NO : PMIOPort  Port=2  Side=Left
  NC : PMIOPort  Port=3  Side=Left
  wires:
  Bus Selector/1 -> Logical Operator/1, Ideal Switch/1  "<b9>"
  C/1 -> Bus Selector/1
  Logical Operator/1 -> Ideal Switch1/1
  connections:
  NC/RConn1 -- Ideal Switch1/LConn1
  NO/RConn1 -- Ideal Switch/LConn1
  Ideal Switch1/RConn1 -- Ideal Switch/RConn1 -- Pole/RConn1

== system sar_adc_3/Circuit Level 12 Bit DAC/DAC_9AB/SPDT_1 ==
  C : Inport
  Bus Selector : BusSelector  OutputSignals=b10
  Ideal Switch : powerlib/Power Electronics/Ideal Switch  Ron=Ron  Lon=0  IC=0  Rs=inf  Cs=0  Measurements=off
  Ideal Switch1 : powerlib/Power Electronics/Ideal Switch  Ron=Ron  Lon=0  IC=0  Rs=inf  Cs=0  Measurements=off
  Logical Operator : Logic  Operator=NOT  AllPortsSameDT=off  OutDataTypeStr=boolean
  Pole : PMIOPort  Side=Right
  NO : PMIOPort  Port=2  Side=Left
  NC : PMIOPort  Port=3  Side=Left
  wires:
  Logical Operator/1 -> Ideal Switch1/1
  C/1 -> Bus Selector/1
  Bus Selector/1 -> Ideal Switch/1, Logical Operator/1  "<b10>"
  connections:
  Pole/RConn1 -- Ideal Switch/RConn1 -- Ideal Switch1/RConn1
  NO/RConn1 -- Ideal Switch/LConn1
  NC/RConn1 -- Ideal Switch1/LConn1

== system sar_adc_3/Circuit Level 12 Bit DAC/DAC_9AB/SPDT_2 ==
  C : Inport
  Bus Selector : BusSelector  OutputSignals=b11
  Ideal Switch : powerlib/Power Electronics/Ideal Switch  Ron=Ron  Lon=0  IC=0  Rs=inf  Cs=0  Measurements=off
  Ideal Switch1 : powerlib/Power Electronics/Ideal Switch  Ron=Ron  Lon=0  IC=0  Rs=inf  Cs=0  Measurements=off
  Logical Operator : Logic  Operator=NOT  AllPortsSameDT=off  OutDataTypeStr=boolean
  Pole : PMIOPort  Side=Right
  NO : PMIOPort  Port=2  Side=Left
  NC : PMIOPort  Port=3  Side=Left
  wires:
  Bus Selector/1 -> Logical Operator/1, Ideal Switch/1  "<b11>"
  C/1 -> Bus Selector/1
  Logical Operator/1 -> Ideal Switch1/1
  connections:
  NC/RConn1 -- Ideal Switch1/LConn1
  NO/RConn1 -- Ideal Switch/LConn1
  Ideal Switch1/RConn1 -- Ideal Switch/RConn1 -- Pole/RConn1

== stateflow chart sar_adc_3/Succesive Approximation Logic ==
  state Idle_Done
    entry: Bit=Nbits-1;
    EOC=1;
    ADC_Out=Dout;
  state Run
    entry: Dout=Dout+2^Bit;
  (junction 52) -> Idle_Done [order 1] : [Bit==0]
  (default) -> Idle_Done
  Idle_Done -> Run : [Start==1]{Dout=-2^Bit;EOC=0;}
  Run -> (junction 52) [order 2] : [Control==0]{Dout=Dout-2^Bit;}
  (junction 52) -> Run [order 2] : [Bit>0]{Bit=Bit-1;}
  Run -> (junction 52) [order 1] : [Control==1]
  data: ADC_Out output int16; EOC output boolean; Start input; Control input; Dout output int16; Bit local double; Nbits input
  events: Clock input RISING_EDGE_EVENT
